simulink model "amp_qam16"  (Simulink 6.0)
settings: Solver=FixedStepDiscrete  StartTime=0.0  StopTime=10  RelTol=1e-3
undefined symbols (not defined in the file or in its folder): Fs, magnitude, read, rfdata
libraries: commsink2 x3, simulink x2, rfports1 x2, commfilt2 x2, commdigbbndam2 x2, rfamplifiers1 x1, dspsnks4 x1, dsparch4 x1, dspsrcs4 x1, commrandsrc2 x1
settings Model: Creator=RobertZ  LastModifiedBy=fwei  ProdHWDeviceType=Specified
settings DataIOCC: SaveOutput=off  SaveTime=off  SignalLoggingName=sigsOut
settings DebuggingCC: CheckExecutionContextPreStartOutputMsg=on  CheckExecutionContextRuntimeOutputMsg=on  SolverPrmCheckMsg=none  InheritedTsInSrcMsg=none
settings HardwareCC: ProdHWDeviceType=Specified
settings ModelReferenceCC: UpdateModelReferenceTargets=IfOutOfDate

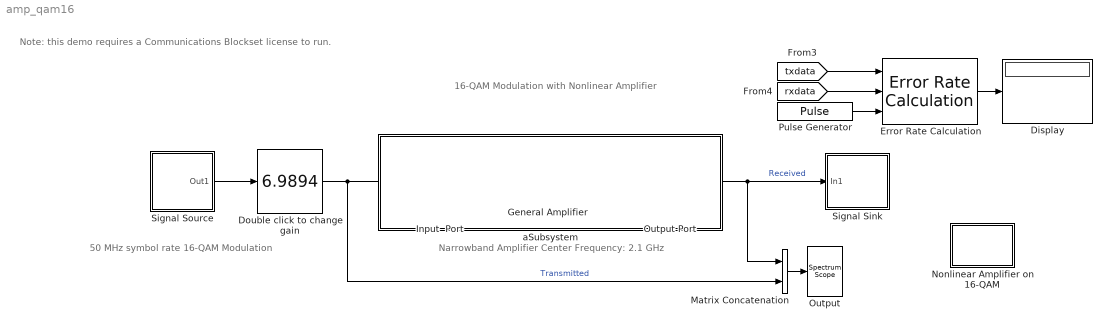
== system amp_qam16 ==
  note: 16-QAM Modulation with Nonlinear Amplifier
  note: 50 MHz symbol rate
      | 16-QAM Modulation
  note: Narrowband Amplifier
      | Center Frequency:  2.1 GHz
  note: Note: this demo requires a
      | Communications Blockset
      | license to run.
  Display : Display
  Double click to change gain : simulink/Math Operations/Slider Gain  low=0.1  gain=6.9894  high=10
  Error Rate Calculation : commsink2/Error Rate Calculation  N=16  st_delay=16*1024  cp_mode=Entire frame  subframe=[]  PMode=Port  WsName=ErrorVec  RsMode2=on  stop=off  numErr=100  maxBits=1e6
  General Amplifier : rfamplifiers1/General Amplifier  PhysicalDomain=rfsystemsdomain  SubClassName=general-amplifier  LeftPortType=p1  RightPortType=p1  LConnTagsString=__newl0  RConnTagsString=__newr0  RFDATA=read(rfdata.data, 'default.amp')  InterpMethod=Linear  IP3Type=OIP3  IIP3=inf  OIP3=inf  NF=0  DisplayData=off  PlotFreq=Derived from Input Port parameters  PlotFreqNoSim=Extracted from RFDATA object  Freq=[1.0e9:1.0e8:2.9e9]  AllPlotType=X-Y plane  NetworkData=S21  PowerData=S11  SmithData=S22  PolarData=S11  ComplexFormat=Magnitude (decibels)  DBFormat=Magnitude (decibels)  PowerFormat=dBm  PhaseFormat=Angle (degrees)  NoneFormat=None
  Input  Port : rfports1/Input Port  Description=source block  MaxLength=128  Fc=2.1e9  Ts=2.5e-9  Zs=50  NoiseFlag=off  seed=67987  GoToTag=BCBGILFOFCAUODBTYHGIPIB
  Matrix Concatenation : simulink/Math Operations/Matrix Concatenation  numInports=2  catMethod=Horizontal
  Nonlinear Amplifier on 16-QAM : Subsystem  PropExecContextAcrossSSBoundary=on
      mask Display: disp('Info')
  Output : dspsnks4/Spectrum Scope  ScopeProperties=on  Domain=Frequency  HorizSpan=1  UseBuffer=off  BufferSize=1024  Overlap=512  inpFftLenInherit=off  FFTlength=1024  numAvg=20  DisplayProperties=off  AxisGrid=on  Memory=off  FrameNumber=on  AxisLegend=on  AxisZoom=off  OpenScopeAtSimStart=on  OpenScopeImmediately=off  FigPos=[311 366 418 221]  AxisProperties=off  XUnits=Hertz  XRange=[-Fs/2...Fs/2]  InheritXIncr=on  XIncr=1.0  XLabel=Samples  YUnits=dB  YLabel=Magnitude, dB  LineProperties=off  LineStyles=-|-  LineMarkers=None  LineColors=[1 0 0]|[0 0 0]
      settings: YMin=-75.3034013425467  YMax=36.8072300077051
  Output Port : rfports1/Output Port  Zl=50  num_Models=3  GoToTag=BCBGILFOFCAUODBTYHGIPIB  DisplayData=off  PlotFreq=Derived from Input Port parameters  Freq=1e9:1e8:3e9  AllPlotType=Composite data  NoBudgetPlot=Composite data  NetworkData=S11  SmithData=S11  PolarData=S11  ComplexFormat=Magnitude (decibels)  DBFormat=Magnitude (decibels)  DBMFormat=dBm  NoneFormat=None
  Pulse Generator : DiscretePulseGenerator  Period=16  SampleTime=1024*2e-8
  Signal Sink : Subsystem  PropExecContextAcrossSSBoundary=on
      mask Display: disp('Signal\nSink')
  Signal Source : Subsystem  PropExecContextAcrossSSBoundary=on
      mask Display: disp('Signal\nSource')
  aSubsystem : Subsystem  PropExecContextAcrossSSBoundary=on
      mask Display: disp('')
  wires:
  Matrix Concatenation/1 -> Output/1
  Output Port/1 -> Signal Sink/1(In1), Matrix Concatenation/1  "Received"
  Signal Source/1(Out1) -> Double click to change gain/1
  Error Rate Calculation/1 -> Display/1
  Pulse Generator/1 -> Error Rate Calculation/3
  [txdata] -> Error Rate Calculation/1
  [rxdata] -> Error Rate Calculation/2
  Double click to change gain/1 -> Input  Port/1, Matrix Concatenation/2  "Transmitted"
  connections:
  Input  Port/RConn1 -- General Amplifier/LConn1
  General Amplifier/RConn1 -- Output Port/LConn1

== system amp_qam16/Nonlinear Amplifier on 16-QAM ==
  note: 16-QAM Modulation with Nonlinear Amplifier
      |
      | This model shows the effect of amplifier nonlinearity on a 16-QAM modulated
      | signal. The 16-QAM constellation is phase rotated and also distorted.
      |
      | The spectrum of the amplifier output also demonstrates spectral regrowth.
      |
      | Double click on the "Gain" block to change the magnitude of the input signal.

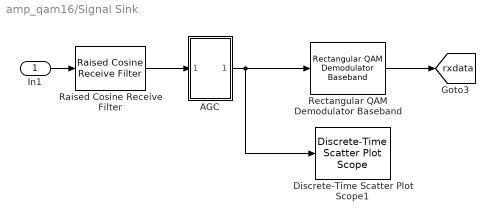
== system amp_qam16/Signal Sink ==
  In1 : Inport  LatchInput=off
  AGC : Subsystem  PropExecContextAcrossSSBoundary=on
      mask Display: disp('AGC');
  Discrete-Time Scatter Plot Scope1 : commsink2/Discrete-Time Scatter Plot Scope  Tag=ScatterPlot  sampPerSymb=8  offsetEye=0  numTraces=800  numNewFrames=800  LineMarkers=.  LineColors=[1 0 0]  fading=on  render=on  AxisGrid=on  xMin=-1.54318163861981  xMax=1.55695676278622  yMin=-1.54272562409615  yMax=1.55741277730988  inphaseLabel=In-phase Amplitude  quadratureLabel=Quadrature Amplitude  openScopeAtSimStart=on  FrameNumber=off  FigPos=[737 311 278 278]  figTitle=Scatter Plot  numLinesMax=8  block_type_=scatter
  Raised Cosine Receive Filter : commfilt2/Raised Cosine Receive Filter  filtType=Square root  N=8  D=4  R=0.2  sampMode=Frame-based  rateMode=Downsampling  downFactor=8  downOffset=0  checkGain=Normalized  filterGain=1  checkCoeff=off  variableName=rcRxFilt  launchFVT=off
  Rectangular QAM Demodulator Baseband : commdigbbndam2/Rectangular QAM Demodulator Baseband  M=16  OutType=Integer  Dec=Binary  PowType=Peak Power  MinDist=2  AvgPow=1  PeakPow=2  Ph=-pi/4  numSamp=1
  tag scope: rxdata=global
  wires:
  Raised Cosine Receive Filter/1 -> AGC/1(In1)
  AGC/1(Out1) -> Rectangular QAM Demodulator Baseband/1, Discrete-Time Scatter Plot Scope1/1
  Rectangular QAM Demodulator Baseband/1 -> [rxdata]
  In1/1 -> Raised Cosine Receive Filter/1

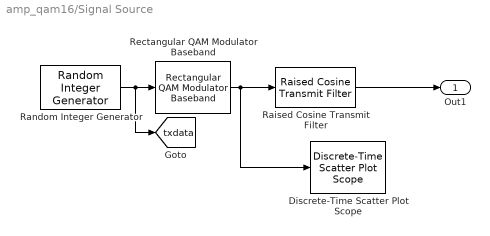
== system amp_qam16/Signal Source ==
  Discrete-Time Scatter Plot Scope : commsink2/Discrete-Time Scatter Plot Scope  Tag=ScatterPlot  sampPerSymb=8  offsetEye=0  numTraces=400  numNewFrames=100  LineMarkers=.  LineColors=[0 0 0]  fading=off  render=on  AxisGrid=on  xMin=-1.5556349186104  xMax=1.56270598642227  yMin=-1.5556349186104  yMax=1.56270598642227  inphaseLabel=In-phase Amplitude  quadratureLabel=Quadrature Amplitude  openScopeAtSimStart=on  FrameNumber=off  FigPos=[4 289 298 298]  figTitle=Scatter Plot  numLinesMax=8  block_type_=scatter
  Raised Cosine Transmit Filter : commfilt2/Raised Cosine Transmit Filter  filtType=Square root  D=4  R=0.2  sampMode=Frame-based  N=8  checkGain=Normalized  filterGain=1  checkCoeff=off  variableName=rcTxFilt  launchFVT=off
  Random Integer Generator : commrandsrc2/Random Integer Generator  mul=16  seed=37  Ts=2e-8  frameBased=on  sampPerFrame=1024  orient=off
  Rectangular QAM Modulator Baseband : commdigbbndam2/Rectangular QAM Modulator Baseband  M=16  InType=Integer  Enc=Binary  PowType=Peak Power  MinDist=2  AvgPow=1  PeakPow=2  Ph=0  numSamp=1
  Out1 : Outport
  tag scope: txdata=global
  wires:
  Random Integer Generator/1 -> Rectangular QAM Modulator Baseband/1, [txdata]
  Rectangular QAM Modulator Baseband/1 -> Raised Cosine Transmit Filter/1, Discrete-Time Scatter Plot Scope/1
  Raised Cosine Transmit Filter/1 -> Out1/1

== system amp_qam16/aSubsystem ==

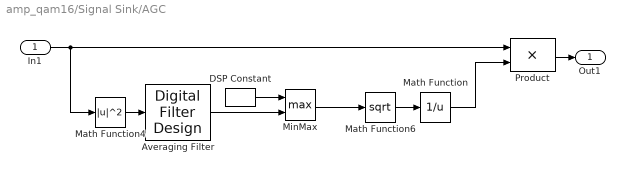
== system amp_qam16/Signal Sink/AGC ==
  In1 : Inport  LatchInput=off
  Averaging Filter : dsparch4/Digital Filter Design
  DSP Constant : dspsrcs4/DSP Constant  Value=eps  SampleMode=Discrete  discreteOutput=Frame-based  continuousOutput=Sample-based  sampTime=-1  framePeriod=-1  dataType=Inherit from 'Constant value'  isSigned=on  wordLen=16  udDataType=sfix(16)  fracBitsMode=Best precision  numFracBits=15  InterpretAs1D=off  Ts=-1  FramebasedOutput=on
      settings: AttributesFormatString=\n\n\n\n
  Math Function : Math  Operator=reciprocal  SaturateOnIntegerOverflow=on
  Math Function4 : Math  Operator=magnitude^2  SaturateOnIntegerOverflow=on
  Math Function6 : Math  Operator=sqrt  SaturateOnIntegerOverflow=on
  MinMax : MinMax  Function=max  Inputs=2  SaturateOnIntegerOverflow=on  InputSameDT=on
  Product : Product  SaturateOnIntegerOverflow=on
  Out1 : Outport
  wires:
  DSP Constant/1 -> MinMax/1
  MinMax/1 -> Math Function6/1
  Averaging Filter/1 -> MinMax/2
  Math Function/1 -> Product/2
  Math Function4/1 -> Averaging Filter/1
  Math Function6/1 -> Math Function/1
  In1/1 -> Product/1, Math Function4/1
  Product/1 -> Out1/1
